simulink model "arduino_serial_gps_standalone"  (R2021b)
settings: Solver=FixedStepAuto  StartTime=0.0  StopTime=10  RelTol=1e-3
PreLoadFcn:
  | addpath(fullfile(fileparts(codertarget.arduinobase.internal.getBaseSpPkgRootDir), 'arduinotarget', 'arduinotargetdemos','demo_src'));
libraries: arduinolib x2, realtime_examples_misc x1
CloseFcn:
  | if (exist('GPSParser.m', 'file') == 2)
  | rmpath(fullfile(fileparts(codertarget.arduinobase.internal.getBaseSpPkgRootDir), 'arduinotarget', 'arduinotargetdemos','demo_src'));
  | end
settings Model: ExtModeTrigDuration=2  ExtModeArchiveDirName=C:\Users\mmordeka\Desktop\2_6_morning  ExtModeAddSuffixToVar=on  Creator=The MathWorks, Inc.  LastModifiedBy=The MathWorks, Inc.
settings SolverCC: AlgebraicLoopSolver=TrustRegion
settings DataIOCC: ReturnWorkspaceOutputs=off
settings OptimizationCC: PassReuseOutputArgsThreshold=0  MaxStackSize=64
settings DebuggingCC: ParameterTunabilityLossMsg=error  SFMachineParentedDataDiag=warning  ArithmeticOperatorsInVariantConditions=warning
settings HardwareCC: ProdBitPerInt=16  ProdBitPerPointer=16  ProdBitPerSizeT=16  ProdBitPerPtrDiffT=16  ProdLargestAtomicFloat=None  ProdWordSize=8  ProdHWDeviceType=Atmel->AVR  UseEmbeddedCoderFeatures=off  UseSimulinkCoderFeatures=off
settings SFSimCC: SimUseLocalCustomCode=off  MATLABDynamicMemAlloc=off  CustomCodeUndefinedFunction=UseInterfaceOnly
settings RTWCC: Description=Embedded Coder  SystemTargetFile=ert.tlc  HardwareBoard=Arduino Mega 2560  TemplateMakefile=ert_default_tmf  GenerateReport=on  RTWUseLocalCustomCode=off  Toolchain=Arduino AVR  BuildConfiguration=Faster Runs  LaunchReport=on
settings CodeAppCC: ForceParamTrailComments=on  OperatorAnnotations=on  StateflowObjectComments=on  MATLABSourceComments=on
settings ERTTargetCC: ERTCustomFileBanners=off  SupportContinuousTime=on  SupportNonInlinedSFcns=on  RemoveResetFunc=off  SupportVariableSizeSignals=on  ModelStepFunctionPrototypeControlCompliant=off

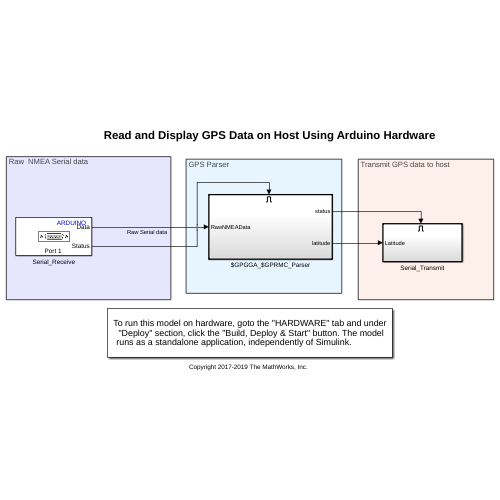
[thumbnail: Simulink's stored preview of the top-level diagram]
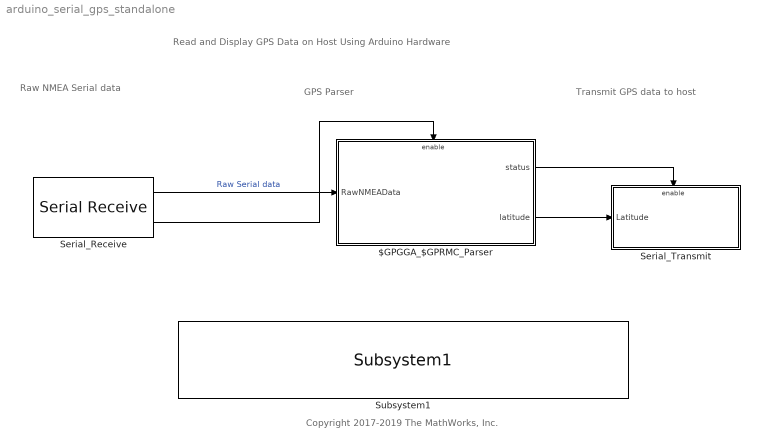
== system arduino_serial_gps_standalone ==
  note: Transmit GPS data to host
  note: GPS Parser
  note: Raw NMEA Serial data
  note: Read and Display GPS Data on Host Using Arduino Hardware
  note: Copyright 2017-2019 The MathWorks, Inc.
  $GPGGA_$GPRMC_Parser : Subsystem  TreatAsAtomicUnit=on
  Serial_Receive : arduinolib/Serial Receive  isARMArch=off  portNumber=1  DataType=uint8  Datalength=32  SampleTime=0.03  showOutStatus=on  blockPlatform=arduino
      settings: SourceProductBaseCode=ARDUINO
  Serial_Transmit : Subsystem
  Subsystem1 : realtime_examples_misc/Subsystem1  SystemSampleTime=-1  VariantActivationTime=update diagram  Latency=0  AutoFrameSizeCalculation=off
      settings: SourceProductBaseCode=SL
  wires:
  Serial_Receive/1 -> $GPGGA_$GPRMC_Parser/1(RawNMEAData)  "Raw Serial data"
  Serial_Receive/2 -> $GPGGA_$GPRMC_Parser/Enable
  $GPGGA_$GPRMC_Parser/1(status) -> Serial_Transmit/Enable
  $GPGGA_$GPRMC_Parser/2(latitude) -> Serial_Transmit/1(Latitude)

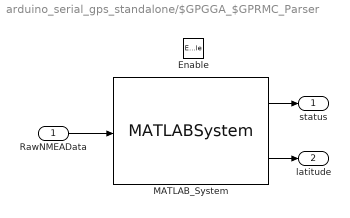
== system arduino_serial_gps_standalone/$GPGGA_$GPRMC_Parser ==
  RawNMEAData : Inport
  Enable : EnablePort  StatesWhenEnabling=reset
  MATLAB_System : MATLABSystem  System=GPSParser  TimeOpt=off  LatOpt=on  LonOpt=off  NoSatOpt=off  HdopOpt=off  AltOpt=off  MslOpt=off  SpeedOpt=off  DateOpt=off  TckAngOpt=off
      mask Type: GPSParser
      mask Display:
      | disp('GPSParser');
      | port_label('input',1,'inData');
      | port_label('output',1,'Status');
      | port_label('output',2,'Latitude');
  status : Outport  OutputWhenDisabled=reset  InitialOutput=0  VectorParamsAs1DForOutWhenUnconnected=off
  latitude : Outport  Port=2  OutputWhenDisabled=reset  InitialOutput=0  VectorParamsAs1DForOutWhenUnconnected=off
  wires:
  MATLAB_System/1 -> status/1
  RawNMEAData/1 -> MATLAB_System/1
  MATLAB_System/2 -> latitude/1

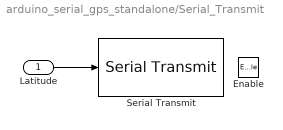
== system arduino_serial_gps_standalone/Serial_Transmit ==
  Latitude : Inport
  Enable : EnablePort
  Serial Transmit : arduinolib/Serial Transmit  portNumber=0  sendmode=println  label=GPS_latitude  sendformat=Decimal  floatprecision=5  blockPlatform=arduino
  wires:
  Latitude/1 -> Serial Transmit/1
